simulink model "Regulator_PI"  (R2022b)
settings: Solver=VariableStepAuto  StartTime=0.0  StopTime=70  RelTol=1e-3
settings Model: Creator=Ioana-Roxana  LastModifiedBy=Ioana-Roxana

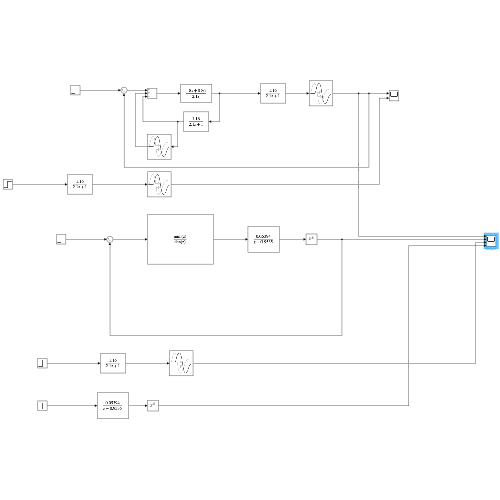
[thumbnail: Simulink's stored preview of the top-level diagram]
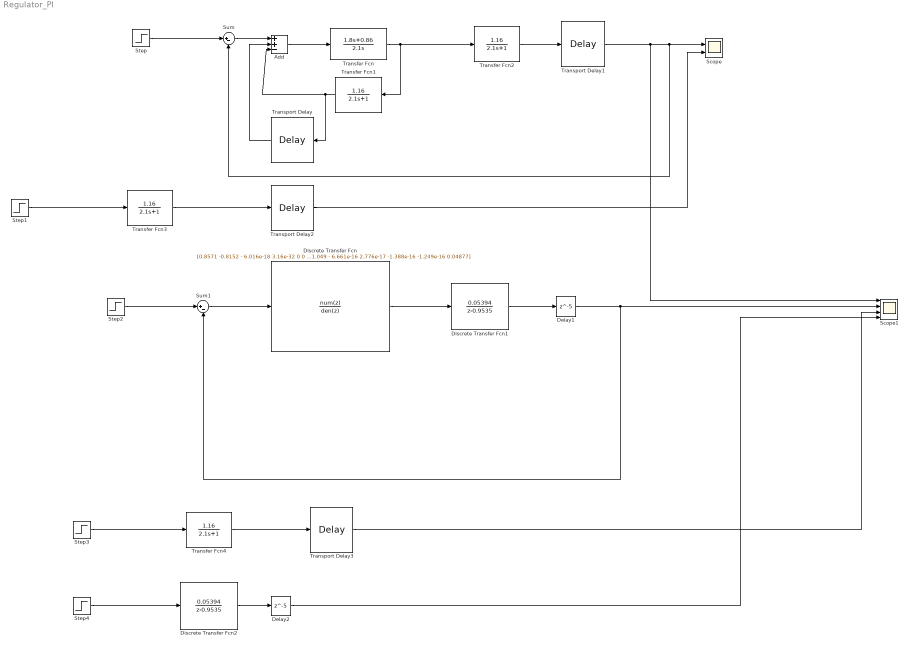
== system Regulator_PI ==
  Add : Sum  Inputs=++-
  Delay1 : Delay  DelayLength=5  SampleTime=0.1
  Delay2 : Delay  DelayLength=5  SampleTime=0.1
  Discrete Transfer Fcn : DiscreteTransferFcn  Numerator=[0.8571 -0.8152 - 6.016e-18 3.16e-32 0 0 0]  Denominator="[1  -1.049 - 6.661e-16 2.776e-17 -1.388e-16 -1.249e-16 0.04877]"  SampleTime=0.1
  Discrete Transfer Fcn1 : DiscreteTransferFcn  Numerator=[0.05394]  Denominator=[1 -0.9535]  SampleTime=0.1
  Discrete Transfer Fcn2 : DiscreteTransferFcn  Numerator=[0.05394]  Denominator=[1 -0.9535]  SampleTime=0.1
  Scope : Scope  NumInputPorts=2
  Scope1 : Scope  NumInputPorts=4
  Step : Step  Time=0  After=120  SampleTime=0
  Step1 : Step  After=137.5  SampleTime=0
  Step2 : Step  Time=0  After=120  SampleTime=0
  Step3 : Step  After=137.5  SampleTime=0
  Step4 : Step  After=137.5  SampleTime=1
  Sum : Sum  Inputs=|+-
  Sum1 : Sum  Inputs=|+-
  Transfer Fcn : TransferFcn  Numerator=[1.8 0.86]  Denominator=[2.1 0]
  Transfer Fcn{1..4} (4 alike) : TransferFcn  Numerator=1.16  Denominator=[2.1 1]
  Transport Delay{,1..3} (4 alike) : TransportDelay  DelayTime=0.5
  wires:
  Step/1 -> Sum/1
  Sum/1 -> Add/1
  Add/1 -> Transfer Fcn/1
  Transfer Fcn/1 -> Transfer Fcn1/1, Transfer Fcn2/1
  Transfer Fcn1/1 -> Transport Delay/1, Add/3
  Transport Delay/1 -> Add/2
  Transfer Fcn2/1 -> Transport Delay1/1
  Transport Delay1/1 -> Scope1/1, Scope/1, Sum/2
  Step1/1 -> Transfer Fcn3/1
  Transfer Fcn3/1 -> Transport Delay2/1
  Transport Delay2/1 -> Scope/2
  Delay1/1 -> Sum1/2, Scope1/2
  Discrete Transfer Fcn1/1 -> Delay1/1
  Step3/1 -> Transfer Fcn4/1
  Discrete Transfer Fcn/1 -> Discrete Transfer Fcn1/1
  Step2/1 -> Sum1/1
  Sum1/1 -> Discrete Transfer Fcn/1
  Transport Delay3/1 -> Scope1/3
  Transfer Fcn4/1 -> Transport Delay3/1
  Step4/1 -> Discrete Transfer Fcn2/1
  Discrete Transfer Fcn2/1 -> Delay2/1
  Delay2/1 -> Scope1/4
